simulink model "wec_model"  (R2012b)
settings: Solver=ode5  StartTime=0.0  StopTime=975  FixedStep=0.025  MaxStep=0.05  RelTol=1e-3
model workspace (MAT data in the model file):
  m = 140076.5
  b_gen = 100000
  Ainf = 151000
  feSeries = [25 25.5 26 26.5 27 27.5 28 28.5 29 29.5 30 30.5 ... (3802 elements, 1901x2)]
  feDt = 0.5
  radIrfDt = 0.05
  radIrfCoeff = [2292.77851319 4575.18487774 4544.13046787 4492.57947507 4420.83993404 4329.34010337 4218.62550272 4089.35514191 3942.2969704 3778.3225815 3598.40121112 3403.59307617 ... (401 elements, 1x401)]
  kHyd = 789737.48825
settings Model: Creator=Brad  LastModifiedBy=Brad

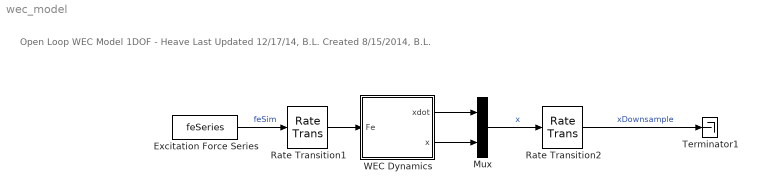
== system wec_model ==
  note: Open Loop WEC Model
      | 1DOF - Heave
      | Last Updated 12/17/14, B.L.
      | Created 8/15/2014, B.L.
  Excitation Force Series : FromWorkspace  VariableName=feSeries  SampleTime=feDt  OutputAfterFinalValue=Setting to zero
  Mux : Mux  Inputs=2
  Rate Transition1 : RateTransition
  Rate Transition2 : RateTransition  OutPortSampleTime=feDt
  Terminator1 : Terminator
  WEC Dynamics : Subsystem
  wires:
  Excitation Force Series/1 -> Rate Transition1/1  "feSim"
  WEC Dynamics/1(xdot) -> Mux/1
  WEC Dynamics/2(x) -> Mux/2
  Mux/1 -> Rate Transition2/1  "x"
  Rate Transition1/1 -> WEC Dynamics/1(Fe)
  Rate Transition2/1 -> Terminator1/1  "xDownsample"

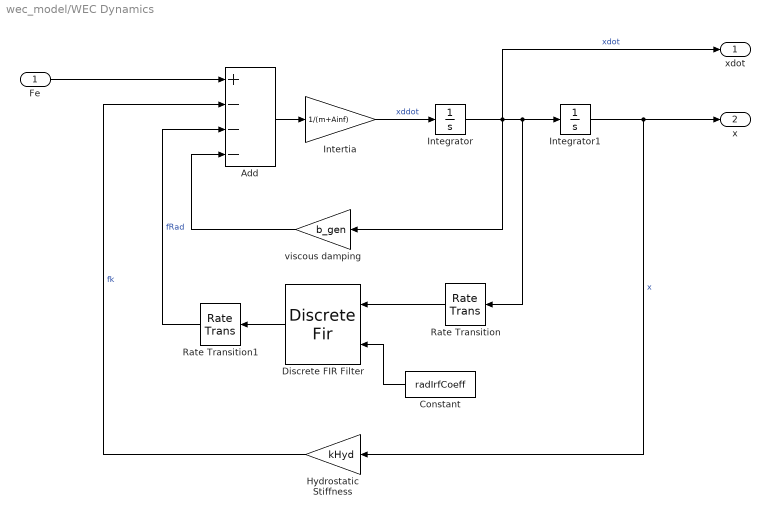
== system wec_model/WEC Dynamics ==
  Fe : Inport
  Add : Sum  Inputs=+---
  Constant : Constant  Value=radIrfCoeff
  Discrete FIR Filter : DiscreteFir  CoefSource=Input port  Coefficients=ones(1, 401)  SampleTime=radIrfDt
  Hydrostatic Stiffness : Gain  Gain=kHyd
  Integrator : Integrator
  Integrator1 : Integrator
  Intertia : Gain  Gain=1/(m+Ainf)
  Rate Transition : RateTransition  OutPortSampleTime=radIrfDt
  Rate Transition1 : RateTransition  OutPortSampleTimeOpt=Inherit
  viscous damping : Gain  Gain=b_gen
  xdot : Outport
  x : Outport  Port=2
  wires:
  Integrator/1 -> viscous damping/1, xdot/1, Rate Transition/1, Integrator1/1  "xdot"
  Fe/1 -> Add/1
  Integrator1/1 -> x/1, Hydrostatic Stiffness/1  "x"
  Hydrostatic Stiffness/1 -> Add/2  "fk"
  Rate Transition/1 -> Discrete FIR Filter/1
  Discrete FIR Filter/1 -> Rate Transition1/1
  Rate Transition1/1 -> Add/3  "fRad"
  Add/1 -> Intertia/1
  Intertia/1 -> Integrator/1  "xddot"
  viscous damping/1 -> Add/4
  Constant/1 -> Discrete FIR Filter/2
